simulink model "PFE"  (R2024a)
settings: Solver=ode23tb  StartTime=0.0  StopTime=inf  RelTol=2e-1
model workspace (MAT data in the model file):
  EngPwr = 352122.842504
  EngWc = 4.047
  Tdiff = 849
  Tlim = 1000
  VEH : object (value not decoded)
libraries: simulink x7, vehdynlibtirecommon x4, autolibutils x4, sim3dlib x3, sharedtransform x2, dspnetwork x2, vehdynlibtire x1, sim3dautolib x1, vehdynlibsteering x1, autolibshared x1
(part 2 of 2)

== system PFE/Powertrain & Driveline/Brakes and Wheels/Veh2Tire/Wheel to Body Transform ==
  VelVeh : Inport  Partition=on  PartitionDimension=2  PartitionWidth=1  PartitionOffset=0
  WhlAng : Inport  Port=2  Partition=on  PartitionDimension=2  PartitionWidth=1  PartitionOffset=0
  Demux1 : Demux  Outputs=3
  Divide1 : Product  Inputs=**  Multiplication=Matrix(*)
  For Each : ForEach  DisableCoverage=on
  Rotation Angles to Direction Cosine Matrix : sharedtransform/Rotation Angles to Direction Cosine Matrix  rotationOrder=ZYX  aMode=2
  Selector : Selector  InputPortWidth=3  IndexOptions=Index vector (dialog)  Indices=[3 2 1]  OutputSizes=1
  xdotWheel : Outport  ConcatenationDimension=1  VectorParamsAs1DForOutWhenUnconnected=off
  ydotWheel : Outport  Port=2  ConcatenationDimension=1  VectorParamsAs1DForOutWhenUnconnected=off
  zdotWheel : Outport  Port=3  ConcatenationDimension=1  VectorParamsAs1DForOutWhenUnconnected=off
  wires:
  Divide1/1 -> Demux1/1
  Demux1/1 -> xdotWheel/1
  Demux1/2 -> ydotWheel/1
  Demux1/3 -> zdotWheel/1
  Rotation Angles to Direction Cosine Matrix/1 -> Divide1/1
  VelVeh/1 -> Divide1/2
  WhlAng/1 -> Selector/1
  Selector/1 -> Rotation Angles to Direction Cosine Matrix/1

== matlab function PFE/MATLAB Function ==
  data: u input; steer output double
function steer = parse_steer(u)
%#codegen
% Parse steering value sent as ASCII text, e.g. "25" or "-40"

steer = double(0);

% Count valid bytes (nonzero)
n = 0;
for i = 1:length(u)
    if u(i) ~= 0
        n = n + 1;
    end
end

if n == 0
    return;
end

% Build character buffer
buf = char(zeros(1, n));
k = 1;
for i = 1:length(u)
    if u(i) ~= 0
        buf(k) = char(u(i));
        k = k + 1;
    end
end

% Convert ASCII text to numeric value
v = str2double(buf);

% Keep only valid real scalar
if ~isnan(v) && isreal(v)
    steer = double(v);
else
    steer = double(0);
end
